simulink model "lab2"  (R2022b)
settings: Solver=VariableStepAuto  StartTime=0.0  StopTime=10.0  RelTol=1e-3
settings Model: Creator=dambi  LastModifiedBy=dambi

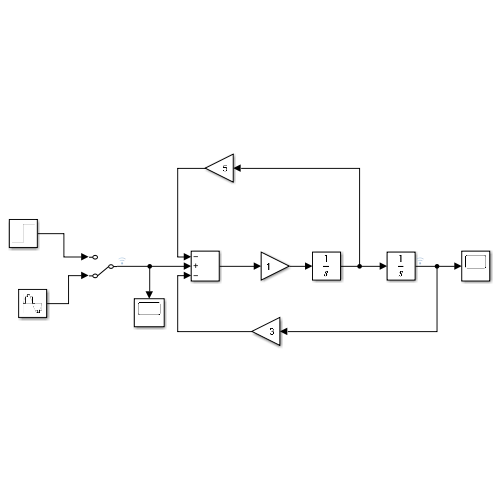
[thumbnail: Simulink's stored preview of the top-level diagram]
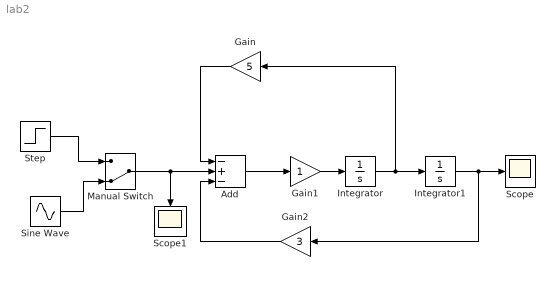
== system lab2 ==
  Add : Sum  Inputs=-+-
  Gain : Gain  Gain=5
  Gain1 : Gain
  Gain2 : Gain  Gain=3
  Integrator : Integrator
  Integrator1 : Integrator
  Manual Switch : ManualSwitch  CurrentSetting=0
  Scope : Scope
  Scope1 : Scope
  Sine Wave : Sin  Frequency=2  SampleTime=0.001
  Step : Step  SampleTime=0
  wires:
  Step/1 -> Manual Switch/1
  Sine Wave/1 -> Manual Switch/2
  Manual Switch/1 -> Scope1/1, Add/2
  Gain/1 -> Add/1
  Gain2/1 -> Add/3
  Add/1 -> Gain1/1
  Gain1/1 -> Integrator/1
  Integrator/1 -> Gain/1, Integrator1/1
  Integrator1/1 -> Gain2/1, Scope/1
